simulink model "test_ibob_data_mux"  (Simulink 6.2)
settings: Solver=ode45  StartTime=0.0  StopTime=3000  RelTol=1e-3
libraries: xbsIndex_r3 x219, xps_library x3
(part 2 of 2)

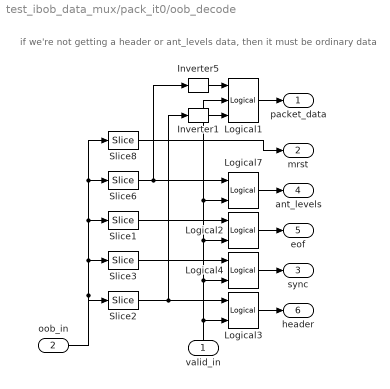
== system test_ibob_data_mux/pack_it0/oob_decode ==
  note: if we're not getting a header or ant_levels data,
      | then it must be ordinary data
  valid_in : Inport  Orientation=up  Port=1  LatchInput=off
  oob_in : Inport  Port=2  LatchInput=off
  Inverter1 : xbsIndex_r3/Inverter  latency=0  explicit_period=off  period=1  en=off  dbl_ovrd=off  show_param=off
      settings: xl_area=[0, 0, 0, 0, 0, 0, 0]
  Inverter5 : xbsIndex_r3/Inverter  latency=0  explicit_period=off  period=1  en=off  dbl_ovrd=off  show_param=off
      settings: xl_area=[0, 0, 0, 0, 0, 0, 0]
  Logical1 : xbsIndex_r3/Logical  logical_function=AND  inputs=3  precision=Full  arith_type=Unsigned  n_bits=8  bin_pt=2  align_bp=on  latency=0  explicit_period=off  period=1  en=off  dbl_ovrd=off  show_param=off
      settings: xl_area=[0, 0, 0, 0, 0, 0, 0]
  Logical{2..4,7} (4 alike) : xbsIndex_r3/Logical  logical_function=AND  inputs=2  precision=Full  arith_type=Unsigned  n_bits=8  bin_pt=2  align_bp=on  latency=0  explicit_period=off  period=1  en=off  dbl_ovrd=off  show_param=off
      settings: xl_area=[0, 0, 0, 0, 0, 0, 0]
  Slice1 : xbsIndex_r3/Slice  mode=Lower Bit Location + Width  nbits=1  bit1=0  base1=MSB of Input  bit0=2  base0=LSB of Input  boolean_output=on  explicit_period=off  period=1  dbl_ovrd=off
  Slice2 : xbsIndex_r3/Slice  mode=Lower Bit Location + Width  nbits=1  bit1=0  base1=MSB of Input  bit0=0  base0=LSB of Input  boolean_output=on  explicit_period=off  period=1  dbl_ovrd=off
  Slice3 : xbsIndex_r3/Slice  mode=Lower Bit Location + Width  nbits=1  bit1=0  base1=MSB of Input  bit0=1  base0=LSB of Input  boolean_output=on  explicit_period=off  period=1  dbl_ovrd=off
  Slice6 : xbsIndex_r3/Slice  mode=Lower Bit Location + Width  nbits=1  bit1=0  base1=MSB of Input  bit0=3  base0=LSB of Input  boolean_output=on  explicit_period=off  period=1  dbl_ovrd=off
  Slice8 : xbsIndex_r3/Slice  mode=Lower Bit Location + Width  nbits=1  bit1=0  base1=MSB of Input  bit0=4  base0=LSB of Input  boolean_output=on  explicit_period=off  period=1  dbl_ovrd=off
  packet_data : Outport
  mrst : Outport  Port=2
  sync : Outport  Port=3
  ant_levels : Outport  Port=4
  eof : Outport  Port=5
  header : Outport  Port=6
  wires:
  Slice8/1 -> mrst/1
  oob_in/1 -> Slice3/1, Slice1/1, Slice6/1, Slice8/1, Slice2/1
  valid_in/1 -> Logical3/2, Logical2/2, Logical7/2, Logical1/2, Logical4/2
  Logical1/1 -> packet_data/1
  Inverter5/1 -> Logical1/1
  Logical7/1 -> ant_levels/1
  Slice1/1 -> Logical2/1
  Logical2/1 -> eof/1
  Slice6/1 -> Logical7/1, Inverter5/1
  Slice2/1 -> Logical3/1, Inverter1/1
  Logical3/1 -> header/1
  Inverter1/1 -> Logical1/3
  Slice3/1 -> Logical4/1
  Logical4/1 -> sync/1

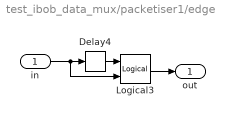
== system test_ibob_data_mux/packetiser1/edge ==
  in : Inport  Port=1  LatchInput=off
  Delay4 : xbsIndex_r3/Delay  latency=1  reg_retiming=off  explicit_period=off  period=1  en=off  accept_only_valid=off  init_zero=on  dbl_ovrd=off  show_param=off
      settings: xl_area=[0, 0, 0, 0, 0, 0, 0]
  Logical3 : xbsIndex_r3/Logical  logical_function=XOR  inputs=2  precision=Full  arith_type=Unsigned  n_bits=8  bin_pt=2  align_bp=on  latency=0  explicit_period=off  period=1  en=off  dbl_ovrd=off  show_param=off
      settings: xl_area=[0, 0, 0, 0, 0, 0, 0]
  out : Outport
  wires:
  in/1 -> Logical3/2, Delay4/1
  Delay4/1 -> Logical3/1
  Logical3/1 -> out/1

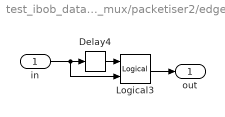
== system test_ibob_data_mux/packetiser2/edge1 ==
  in : Inport  Port=1  LatchInput=off
  Delay4 : xbsIndex_r3/Delay  latency=1  reg_retiming=off  explicit_period=off  period=1  en=off  accept_only_valid=off  init_zero=on  dbl_ovrd=off  show_param=off
      settings: xl_area=[0, 0, 0, 0, 0, 0, 0]
  Logical3 : xbsIndex_r3/Logical  logical_function=XOR  inputs=2  precision=Full  arith_type=Unsigned  n_bits=8  bin_pt=2  align_bp=on  latency=0  explicit_period=off  period=1  en=off  dbl_ovrd=off  show_param=off
      settings: xl_area=[0, 0, 0, 0, 0, 0, 0]
  out : Outport
  wires:
  Logical3/1 -> out/1
  Delay4/1 -> Logical3/1
  in/1 -> Delay4/1, Logical3/2
